simulink model "FirstAttempt_Enceladus"  (R2018b)
settings: Solver=VariableStepAuto  StartTime=0.0  StopTime=time  RelTol=1e-3
values from neighbouring files (symbols this model uses):
  A_side = 2 * A_front    (= 0.02)    [MultipleNodes.m]    (also in OneNode.m)
  eps_f = 1    [OneNode.m]
  eps_l = 0.81    [OneNode.m]
  Qa = 0    [OneNode.m]
  Qasat = 0    [OneNode.m]
  Qi = 0.2*Qdiss    (= 0.6)    [OneNode.m]
  Qir = Wir*A_front *eps_b*REF    (= 1.4821904091e-05)    [OneNode.m]
  Qirsat = 0    [OneNode.m]
  QS = 0    [OneNode.m]
  sigma = 5.67e-8    (= 5.67e-08)    [MultipleNodes.m]    (also in OneNode.m)
  Tds = 4    [MultipleNodes.m]    (also in OneNode.m)
  Tsc_h = T_sc(1,2)    [OneNode.m]
libraries: fl_lib x23, nesl_utility x10
settings Model: Creator=aloisia  LastModifiedBy=aloisia

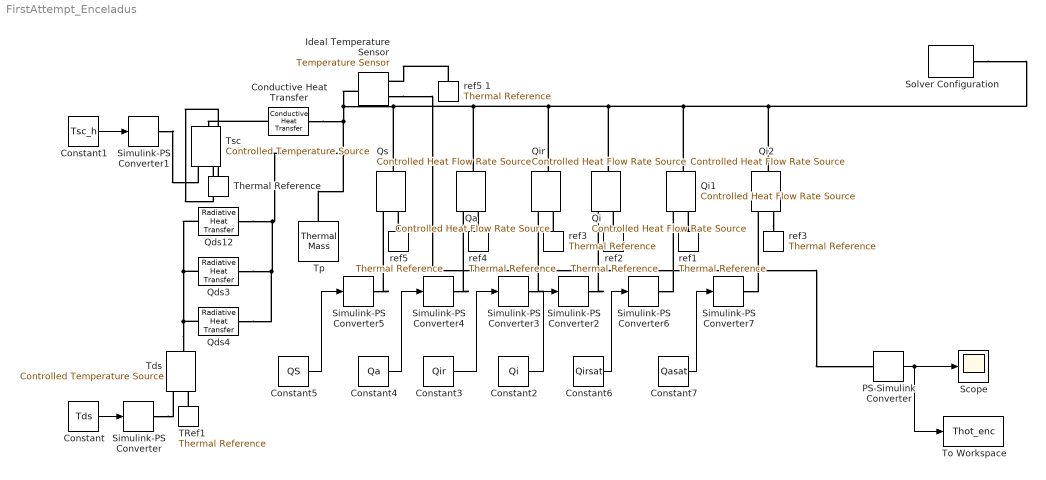
== system FirstAttempt_Enceladus ==
  Conductive Heat Transfer : fl_lib/Thermal/Thermal Elements/Conductive Heat Transfer  area=0.005 m^2  thickness=0.01 m  th_cond=Gsc W/(m*K)  T_specify=off  T_priority=None  T=0 K  T_nominal_specify=off  T_nominal_unit=K  T_nominal_value=1  Q_specify=off  Q_priority=None  Q=0 J/s  Q_nominal_specify=off  Q_nominal_unit=W  Q_nominal_value=1
      settings: SourceProductName=Simscape
  Constant : Constant  Value=Tds
  Constant1 : Constant  Value=Tsc_h
  Constant2 : Constant  Value=Qi
  Constant3 : Constant  Value=Qir
  Constant4 : Constant  Value=Qa
  Constant5 : Constant  Value=QS
  Constant6 : Constant  Value=Qirsat
  Constant7 : Constant  Value=Qasat
  Ideal Temperature Sensor : fl_lib/Thermal/Thermal Sensors/Temperature Sensor
  PS-Simulink Converter : nesl_utility/PS-Simulink Converter  PhysicalDomain=network_engine_domain  SubClassName=ps_output  LeftPortType=input  RightPortType=output  PseudoPeriodic=off  Frequencies=[]  Unit=1  AffineConversion=off
  Qa : fl_lib/Thermal/Thermal Sources/Controlled Heat Flow Rate Source
      settings: SourceProductName=Simscape
  Qds12 : fl_lib/Thermal/Thermal Elements/Radiative Heat Transfer  area=2*A_side m^2  rad_tr_coeff=sigma*eps_l W/(m^2*K^4)  T_specify=off  T_priority=None  T=0 K  T_nominal_specify=off  T_nominal_unit=K  T_nominal_value=1  Q_specify=off  Q_priority=None  Q=0 J/s  Q_nominal_specify=off  Q_nominal_unit=W  Q_nominal_value=1
      settings: SourceProductName=Simscape  SourceProductBaseCode=SS
  Qds3 : fl_lib/Thermal/Thermal Elements/Radiative Heat Transfer  area=A_front m^2  rad_tr_coeff=sigma*eps_f W/(m^2*K^4)  T_specify=off  T_priority=None  T=0 K  T_nominal_specify=off  T_nominal_unit=K  T_nominal_value=1  Q_specify=off  Q_priority=None  Q=0 J/s  Q_nominal_specify=off  Q_nominal_unit=W  Q_nominal_value=1
      settings: SourceProductName=Simscape  SourceProductBaseCode=SS
  Qds4 : fl_lib/Thermal/Thermal Elements/Radiative Heat Transfer  area=A_front m^2  rad_tr_coeff=sigma*eps_f W/(m^2*K^4)  T_specify=off  T_priority=None  T=0 K  T_nominal_specify=off  T_nominal_unit=K  T_nominal_value=1  Q_specify=off  Q_priority=None  Q=0 J/s  Q_nominal_specify=off  Q_nominal_unit=W  Q_nominal_value=1
      settings: SourceProductName=Simscape  SourceProductBaseCode=SS
  Qi : fl_lib/Thermal/Thermal Sources/Controlled Heat Flow Rate Source
      settings: SourceProductName=Simscape
  Qi1 : fl_lib/Thermal/Thermal Sources/Controlled Heat Flow Rate Source
      settings: SourceProductName=Simscape
  Qi2 : fl_lib/Thermal/Thermal Sources/Controlled Heat Flow Rate Source
      settings: SourceProductName=Simscape
  Qir : fl_lib/Thermal/Thermal Sources/Controlled Heat Flow Rate Source
      settings: SourceProductName=Simscape
  Qs : fl_lib/Thermal/Thermal Sources/Controlled Heat Flow Rate Source
      settings: SourceProductName=Simscape
  Scope : Scope
  Simulink-PS Converter{,1..7} (8 alike) : nesl_utility/Simulink-PS Converter  PhysicalDomain=network_engine_domain  SubClassName=ps_input  LeftPortType=input  RightPortType=output  PseudoPeriodic=off  Frequencies=[]  NoiseDistribution=none  NoiseParameters=[]  Unit=1  AffineConversion=off  FilteringAndDerivatives=zero  SimscapeFilterOrder=1  InputFilterTimeConstant=0.001  UdotUserProvided=1
  Solver Configuration : nesl_utility/Solver Configuration  PhysicalDomain=network_engine_domain  SubClassName=solver  LeftPortType=input  RightPortType=generic  Tones=[]  Harmonics=[]  SimulateNoise=off  Profile=off  UseLocalSampling=off  EnableSwitchedLinearOptims=on  FrequencyDomain=off  UseCCode=off  RelTol=0.001  AbsTol=1e-06  MinStep=1e-09  ToWorkspace=off  RevertToSquareIcSolve=off  NumHomotopyIterations=100  PhasorMode=off  PhasorModeNumHarmonics=1  DoDC=off  ResidualTolerance=1e-09  UseLocalSolver=off  LocalSolverChoice=NE_BACKWARD_EULER_ADVANCER  LocalSolverSampleTime=0.001  DoFixedCost=off  MaxNonlinIter=3  MaxModeIter=2  LinearAlgebra=Full  EquationFormulation=NE_TIME_EF  DelaysMemoryBudget=1024  AutomaticFiltering=on  FilteringTimeConstant=0.0001  PartitionStorageMethod=AS_NEEDED  PartitionMemoryBudget=1024
  TRef1 : fl_lib/Thermal/Thermal Elements/Thermal Reference
  Tds : fl_lib/Thermal/Thermal Sources/Controlled Temperature Source
      settings: SourceProductName=Simscape
  Thermal Reference : fl_lib/Thermal/Thermal Elements/Thermal Reference
  To Workspace : ToWorkspace  VariableName=Thot_enc  SaveFormat=Timeseries  SampleTime=-1
  Tp : fl_lib/Thermal/Thermal Elements/Thermal Mass  mass=5 kg  sp_heat=447 J/kg/K  T_specify=on  T_priority=High  T=287.15 K  T_nominal_specify=off  T_nominal_unit=K  T_nominal_value=1  Q_specify=off  Q_priority=None  Q=0 J/s  Q_nominal_specify=off  Q_nominal_unit=W  Q_nominal_value=1
  Tsc : fl_lib/Thermal/Thermal Sources/Controlled Temperature Source
      settings: SourceProductName=Simscape
  ref{1..4} (4 alike) : fl_lib/Thermal/Thermal Elements/Thermal Reference
  "ref3 " : fl_lib/Thermal/Thermal Elements/Thermal Reference
  "ref5 " : fl_lib/Thermal/Thermal Elements/Thermal Reference
  ref5 1 : fl_lib/Thermal/Thermal Elements/Thermal Reference
  wires:
  Constant4/1 -> Simulink-PS Converter4/1
  Constant5/1 -> Simulink-PS Converter5/1
  Constant1/1 -> Simulink-PS Converter1/1
  PS-Simulink Converter/1 -> To Workspace/1, Scope/1
  Constant/1 -> Simulink-PS Converter/1
  Constant2/1 -> Simulink-PS Converter2/1
  Constant3/1 -> Simulink-PS Converter3/1
  Constant6/1 -> Simulink-PS Converter6/1
  Constant7/1 -> Simulink-PS Converter7/1
  connections:
  Tds/LConn1 -- Qds12/LConn1 -- Qds3/LConn1 -- Qds4/LConn1
  Qds3/RConn1 -- Conductive Heat Transfer/RConn1 -- Ideal Temperature Sensor/LConn1 -- Qi2/LConn1 -- Solver Configuration/RConn1 -- Qi1/LConn1 -- Qi/LConn1 -- Qir/LConn1 -- Qa/LConn1 -- Qs/LConn1 -- Tp/LConn1 -- Qds12/RConn1 -- Qds4/RConn1
  Simulink-PS Converter3/RConn1 -- Qir/RConn1
  "ref5 "/LConn1 -- Qs/RConn2
  Conductive Heat Transfer/LConn1 -- Tsc/LConn1
  "ref3 "/LConn1 -- Qir/RConn2
  ref5 1/LConn1 -- Ideal Temperature Sensor/RConn1
  Ideal Temperature Sensor/RConn2 -- PS-Simulink Converter/LConn1
  Simulink-PS Converter4/RConn1 -- Qa/RConn1
  Simulink-PS Converter5/RConn1 -- Qs/RConn1
  Simulink-PS Converter2/RConn1 -- Qi/RConn1
  ref2/LConn1 -- Qi/RConn2
  TRef1/LConn1 -- Tds/RConn2
  Simulink-PS Converter/RConn1 -- Tds/RConn1
  Thermal Reference/LConn1 -- Tsc/RConn2
  ref4/LConn1 -- Qa/RConn2
  Simulink-PS Converter6/RConn1 -- Qi1/RConn1
  ref1/LConn1 -- Qi1/RConn2
  Simulink-PS Converter7/RConn1 -- Qi2/RConn1
  Qi2/RConn2 -- ref3/LConn1
  Simulink-PS Converter1/RConn1 -- Tsc/RConn1
